simulink model "motor_model_23b_controller"  (R2025b)
settings: Solver=VariableStepAuto  StartTime=0.0  StopTime=sim_time  RelTol=1e-3
values from neighbouring files (symbols this model uses):
  D = 8.57e-7    (= 8.57e-07)    [motor_model_m.m]    (also in sampling_exercise.m)
  final_step_value = 100    [motor_model_m.m]
  J = 0.94e-6    (= 9.4e-07)    [motor_model_m.m]    (also in sampling_exercise.m)
  K_P = 0.013    [motor_model_m.m]
  Kb = Kt    (= 0.008863)    [motor_model_m.m]    (also in sampling_exercise.m)
  Kt = 0.008863    [motor_model_m.m]    (also in sampling_exercise.m)
  L = 3.57e-3    (= 0.00357)    [motor_model_m.m]    (also in sampling_exercise.m)
  R = 3.57    [motor_model_m.m]    (also in sampling_exercise.m)
  r2m = wheelRadius/gear    (= 0.00309917355372)    [motor_model_m.m]    (also in sampling_exercise.m = 0.003125)
  sat_lower_limit = -8    [motor_model_m.m]
  sat_upper_limit = 8    [motor_model_m.m]
  step_time = 0.1    [motor_model_m.m]
  tau_I = 0.04    [motor_model_m.m]
  time_delay = 0.01    [motor_model_m.m]
settings Model: Creator=chr  LastModifiedBy=migue

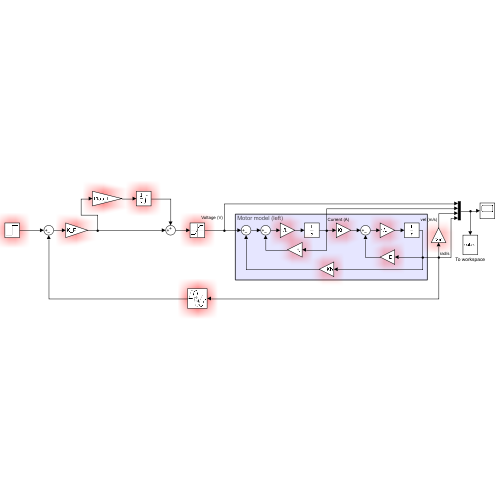
[thumbnail: Simulink's stored preview of the top-level diagram]
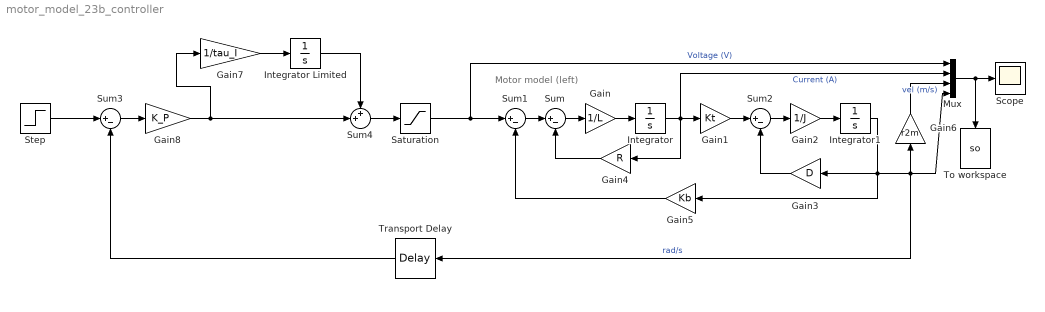
== system motor_model_23b_controller ==
  note: Motor model (left)
  Gain : Gain  Gain=1/L
  Gain1 : Gain  Gain=Kt
  Gain2 : Gain  Gain=1/J
  Gain3 : Gain  Gain=D
  Gain4 : Gain  Gain=R
  Gain5 : Gain  Gain=Kb
  Gain6 : Gain  Gain=r2m
  Gain7 : Gain  Gain=1/tau_I
  Gain8 : Gain  Gain=K_P
  Integrator : Integrator
  Integrator Limited : Integrator  LimitOutput=on  UpperSaturationLimit=sat_upper_limit  LowerSaturationLimit=sat_lower_limit
  Integrator1 : Integrator
  Mux : Mux
  Saturation : Saturate  UpperLimit=sat_upper_limit  LowerLimit=sat_lower_limit
  Scope : Scope
      settings: ActiveDisplayYMinimum=-0.28935  ActiveDisplayYMaximum=6.07084
  Step : Step  Time=step_time  After=final_step_value  SampleTime=0
  Sum{,1..3} (4 alike) : Sum  Inputs=|+-
  Sum4 : Sum  Inputs=++|
  To workspace : ToWorkspace  VariableName=so  SaveFormat=Timeseries  SampleTime=-1
  Transport Delay : TransportDelay  DelayTime=time_delay
  wires:
  Gain/1 -> Integrator/1
  Sum/1 -> Gain/1
  Integrator/1 -> Mux/2, Gain4/1, Gain1/1  "Current (A)"
  Sum1/1 -> Sum/1
  Gain1/1 -> Sum2/1
  Sum2/1 -> Gain2/1
  Gain2/1 -> Integrator1/1
  Integrator1/1 -> Gain3/1, Gain5/1, Transport Delay/1, Gain6/1, Mux/4  "rad/s"
  Gain3/1 -> Sum2/2
  Gain4/1 -> Sum/2
  Gain5/1 -> Sum1/2
  Mux/1 -> Scope/1, To workspace/1
  Gain6/1 -> Mux/3  "vel (m/s)"
  Saturation/1 -> Sum1/1, Mux/1  "Voltage (V)"
  Step/1 -> Sum3/1
  Sum3/1 -> Gain8/1
  Sum4/1 -> Saturation/1
  Gain7/1 -> Integrator Limited/1
  Integrator Limited/1 -> Sum4/1
  Gain8/1 -> Sum4/2, Gain7/1
  Transport Delay/1 -> Sum3/2
